simulink model "rispostaAdIngressi"  (R2023a)
settings: Solver=ode4  StartTime=0.0  StopTime=50  FixedStep=0.001  RelTol=1e-3
model workspace (MAT data in the model file):
  s = tf
  s.IOSize_ = [1 1]
  s.Data_ = ltipack.tfdata
  s.Data_.num = {[1 0]}
  s.Data_.den = {[0 1]}
  s.Data_.Delay.Input = 0
  s.Data_.Delay.Output = 0
  s.Data_.Delay.IO = 0
  s.Data_.Ts = 0
libraries: simulink x1
settings Model: Creator=Manuele  LastModifiedBy=Manuele

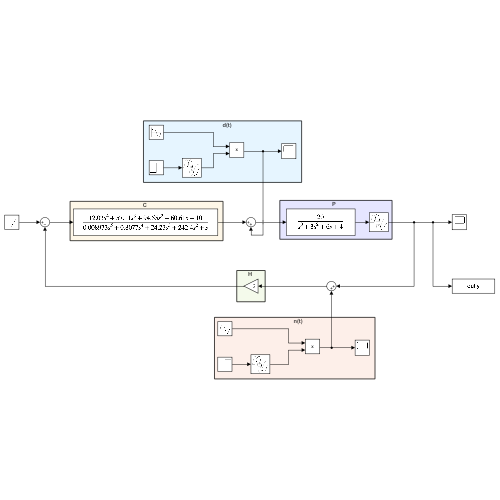
[thumbnail: Simulink's stored preview of the top-level diagram]
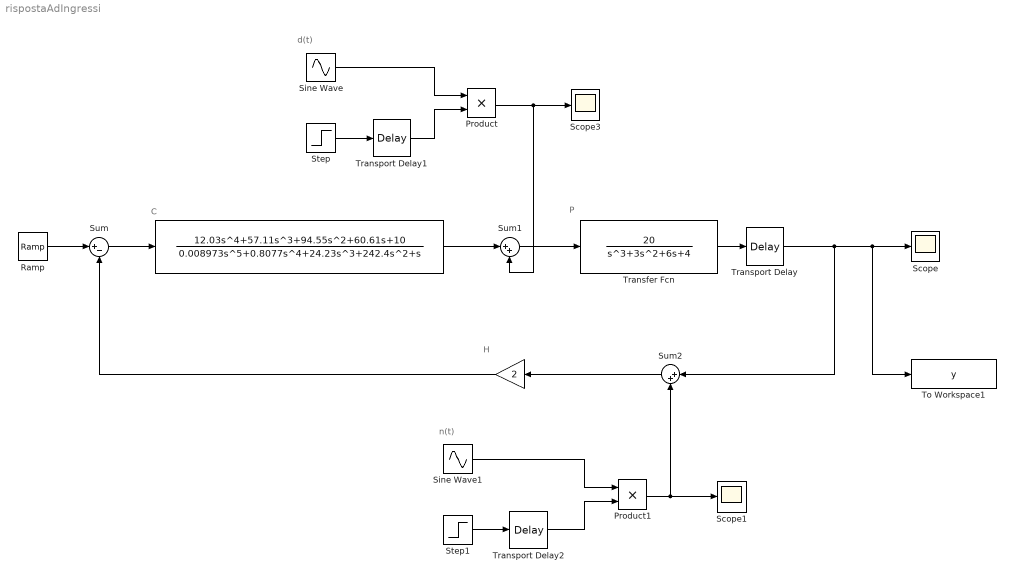
== system rispostaAdIngressi ==
  note: d(t)
  note: C
  note: P
  note: n(t)
  note: H
  " " : TransferFcn  Numerator=[12.03 57.11 94.55 60.61 10]  Denominator=[0.008973 0.8077 24.23 242.4 1 0]
  "   " : Gain  Gain=2
  Product : Product
  Product1 : Product
  Ramp : simulink/Sources/Ramp  slope=2  start=0  InitialOutput=0
  Scope : Scope
  Scope1 : Scope
  Scope3 : Scope
  Sine Wave : Sin  Frequency=0.02  SampleTime=0
  Sine Wave1 : Sin  Frequency=50  SampleTime=0
  Step : Step  Time=0  Before=1  SampleTime=0
  Step1 : Step  Time=0  Before=1  SampleTime=0
  Sum : Sum  Inputs=|+-
  Sum1 : Sum  Inputs=|++
  Sum2 : Sum  Inputs=|++
  To Workspace1 : ToWorkspace  VariableName=y  SaveFormat=Timeseries  SampleTime=-1
  Transfer Fcn : TransferFcn  Numerator=[20]  Denominator=[1 3 6 4]
  Transport Delay : TransportDelay  DelayTime=0.1
  Transport Delay1 : TransportDelay  DelayTime=20
  Transport Delay2 : TransportDelay  DelayTime=40
  wires:
  "   "/1 -> Sum/2
  Sum/1 -> " "/1
  Ramp/1 -> Sum/1
  " "/1 -> Sum1/1
  Transfer Fcn/1 -> Transport Delay/1
  Sum1/1 -> Transfer Fcn/1
  Transport Delay/1 -> Sum2/1, To Workspace1/1, Scope/1
  Product/1 -> Sum1/2, Scope3/1
  Step/1 -> Transport Delay1/1
  Sine Wave/1 -> Product/1
  Transport Delay1/1 -> Product/2
  Step1/1 -> Transport Delay2/1
  Sine Wave1/1 -> Product1/1
  Transport Delay2/1 -> Product1/2
  Product1/1 -> Scope1/1, Sum2/2
  Sum2/1 -> "   "/1
